simulink model "Main_bikesim_ontest2"  (R2024b)
settings: Solver=FixedStepAuto  StartTime=0.0  StopTime=inf  FixedStep=0.0005
values from neighbouring files (symbols this model uses):
  A_d = permute(A_d,[1,3,2])    [Main_sim.m]    (also in Startup_labview_v2.m; sensor_error_test_sequence.m = (eye(size(A))+Ts*A))
  Ad_t = eye(1)+Ts*A_t    [Main_sim.m]    (also in Startup_labview_v2.m = (eye(size(A_t))+Ts*A_t))
  B_d = zeros(V_n,7,1)    [Main_sim.m]    (also in Startup_labview_v2.m; sensor_error_test_sequence.m = Ts*B)
  badGPS = 0    [Main_sim.m]
  Bd_t = B_t*Ts    [Main_sim.m]    (also in Startup_labview_v2.m)
  bike_model = 1    [Main_sim.m]
  bike_params = LoadBikeParameters(bike)    [Compare_real_to_sim.m]    (also in MPC_Data_train.m = LoadBikeParameters("green"); Main_sim.m; Startup_labview_v2.m; sensor_error_test_sequence.m)
  C = mpc_outer_params.Cd    [MPC_Data_train.m]    (also in Main_sim.m = permute(C,[1,3,2]); Startup_labview_v2.m = permute(C,[1,3,2]); fromIMU2trajectory.m = (W_roll * W_roll.') / max(1, size(W_roll,2)); sensor_data_check.m = (W_roll * W_roll.') / max(1, size(W_roll,2)))
  C_t = zeros(V_n,1)    [Main_sim.m]    (also in Startup_labview_v2.m)
  counter = zeros(V_n,1)    [Main_sim.m]    (also in Startup_labview_v2.m; sensor_error_test_sequence.m = 9)
  D = mpc_outer_params.Dd    [MPC_Data_train.m]    (also in Main_sim.m = zeros(V_n,7,1); Startup_labview_v2.m = zeros(V_n,7,1))
  D_t = zeros(V_n,1)    [Main_sim.m]    (also in Startup_labview_v2.m)
  e1_max = abs(-k2*e2_max/k1)    [Startup_labview_v2.m]
  friction_coefficient = 0.004    [Main_sim.m]
  gg = 9.81    [Main_sim.m]    (also in Startup_labview_v2.m)
  hor_dis = 5    [Main_sim.m]
  I_balancing_outer = 0.0    (= 0)    [Main_sim.m]    (also in Startup_labview_v2.m; sensor_error_test_sequence.m)
  indoor = 0    [Main_sim.m]
  initial_state_estimate = initial_state    [Main_sim.m]    (also in sensor_error_test_sequence.m)
  interpolation = 0    [Main_sim.m]
  k1 = K(1)    [Startup_labview_v2.m]
  k2 = K(2)    [Startup_labview_v2.m]
  K_GPS = permute(K_GPS,[1,3,2])    [Main_sim.m]    (also in Startup_labview_v2.m)
  K_noGPS = permute(K_noGPS,[1,3,2])    [Main_sim.m]    (also in Startup_labview_v2.m)
  lambda = bike_params.lambda    [MPC_Data_train.m]    (also in sensor_error_test_sequence.m = bike_params.lambda_mod)
  lf = bike_params.lf    [MPC_Data_train.m]    (also in sensor_error_test_sequence.m = bike_params.lf_mod)
  linearizedMatrices = [Ad_t, Bd_t, C_t, D_t, V']    [Main_sim.m]
  lr = bike_params.lr    [MPC_Data_train.m]    (also in sensor_error_test_sequence.m = bike_params.lr_mod)
  P_balancing_inner = 3.5    [Main_sim.m]    (also in Startup_labview_v2.m; sensor_error_test_sequence.m)
  P_balancing_outer = 3.75    [Main_sim.m]    (also in Startup_labview_v2.m; sensor_error_test_sequence.m)
  psiref = zeros(length(Xref), 1)    [Refgeneration_test.m]
  ref_dis = 1    [Main_sim.m]    (also in differenttest.m = 0.8; differenttest_Simon.m = 0.1)
  T = [ 1,  sin(phi)*tan(th),  cos(phi)*tan(th) ... (first row only)    [Copy_of_fromIMU2trajectory.m]    (also in Main_sim.m = TransMatrix(bike_params); fromIMU2trajectory.m; sensor_error_test_sequence.m = Rz*Ry*Rx; shorttrajectory.m = table(Xref, Yref, Psiref, Vref, t, 'VariableNames', {'Xref',)
  t_ref = equal_distances / speed    [differenttest.m]    (also in differenttest_Simon.m = linspace(0, (lL-1)/Vref_test, lL)')
  Ts = 0.01    [Main_sim.m]    (also in Startup_labview_v2.m; sensor_error_test_sequence.m)
  V = round(V,1)    [Main_sim.m]    (also in Startup_labview_v2.m)
  v_init = Vref(1)    [Main_sim.m]    (also in Startup_labview_v2.m)
  Vref = zeros(length(Xref), 1)    [Refgeneration_test.m]    (also in differenttest.m = Vref_test * ones(N_line, 1); differenttest_Simon.m = Vref_test * ones(N_line, 1))
  vv = 2.6    [Main_sim.m]    (also in Refgeneration.m = table_ref.v)
  Xref = [Xref;Xref2]    [ReferenceGenerator.m]    (also in concatenate.m; differenttest.m = Xref(:); differenttest_Simon.m = interp1(s, x_path, s_eq, 'linear')')
  Yref = [Yref;Yref2]    [ReferenceGenerator.m]    (also in concatenate.m; differenttest.m = Yref(:); differenttest_Simon.m = interp1(s, y_path, s_eq, 'linear')')
undefined symbols (not defined in the file or in its folder): initial_state, pert_deltadot_state, pert_deltadot_state_fun, pert_phidot_state, pert_phidot_state_fun
libraries: simulink x11, slpidlib x4, matrix_library x1, eeGeneralControl x1
(part 2 of 2)

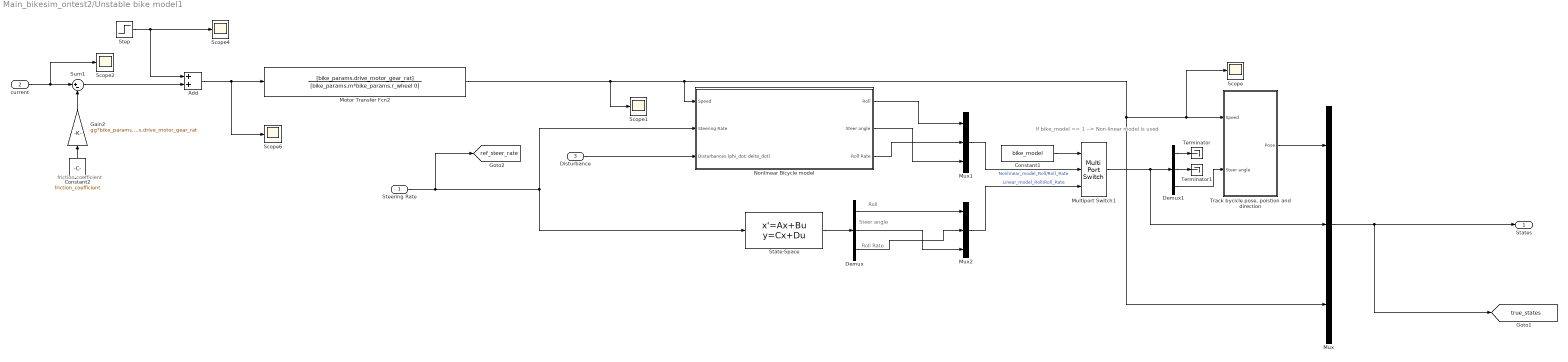
== system Main_bikesim_ontest2/Unstable bike model1 ==
  note: Steer angle
  note: Roll Rate
  note: Roll
  note: If bike_model == 1 --> Non-linear model is used
  note: friction coefficient
  Steering Rate : Inport
  current : Inport  Port=2
  Disturbance : Inport  Port=3
  Add : Sum
  Constant1 : Constant  Value=bike_model
  Constant2 : Constant  Value=friction_coefficient
  Demux : Demux  Outputs=3
  Demux1 : Demux  Outputs=3
  Gain2 : Gain  Gain=gg*bike_params.m*bike_params.r_wheel/bike_params.drive_motor_gear_rat
  Motor Transfer Fcn2 : TransferFcn  Numerator=[bike_params.drive_motor_gear_rat]  Denominator=[bike_params.m*bike_params.r_wheel 0]
  Multiport Switch1 : MultiPortSwitch  Inputs=2  SaturateOnIntegerOverflow=off  InputSameDT=off
  Mux : Mux  Inputs=3
  Mux1 : Mux  Inputs=3
  Mux2 : Mux  Inputs=3
  Nonlinear Bicycle model : Subsystem
  Scope{,1..2,4,6} (5 alike) : Scope
  State-Space : StateSpace  A=[0 0 1; 0 0 0 ; gg/bike_params.h (vv^2/bike_params.h-(gg*bike_params.lr*bike_params.c/(bike_params.h^2*(bike_params.lr+bike_params.lf))))*sin(bike_params.lambda) 0]  B=[0; 1 ; bike_params.lr*vv/((bike_params.lr+bike_params.lf)*bike_params.h)]  C=[1 0 0; 0 1 0 ; 0 0 1]  D=[0;0;0]  InitialCondition=[0; 0 ; 0]
  Step : Step  Time=10  After=0  SampleTime=5
  Sum1 : Sum  Inputs=|+-
  Terminator : Terminator
  Terminator1 : Terminator
  "Track bycicle pose, poistion and direction" : Subsystem
  States : Outport
  tag scope: ref_steer_rate=global, true_states=global
  wires:
  Steering Rate/1 -> State-Space/1, Nonlinear Bicycle model/2(Steering Rate), [ref_steer_rate]
  Nonlinear Bicycle model/3(Roll Rate) -> Mux1/2
  Nonlinear Bicycle model/2(Steer angle) -> Mux1/3
  Demux/1 -> Mux2/1
  Demux/3 -> Mux2/2
  Mux1/1 -> Multiport Switch1/2  "Nonlinear_model_Roll/Roll_Rate"
  Mux2/1 -> Multiport Switch1/3  "Linear_model_Roll/Roll_Rate"
  Constant1/1 -> Multiport Switch1/1
  Disturbance/1 -> Nonlinear Bicycle model/3(Disturbances (phi_dot; delta_dot))
  "Track bycicle pose, poistion and direction"/1(Pose) -> Mux/1
  Mux/1 -> States/1, [true_states]
  Nonlinear Bicycle model/1(Roll) -> Mux1/1
  State-Space/1 -> Demux/1
  Demux/2 -> Mux2/3
  Multiport Switch1/1 -> Mux/2, Demux1/1
  Demux1/3 -> "Track bycicle pose, poistion and direction"/2(Steer angle)
  Demux1/1 -> Terminator/1
  Demux1/2 -> Terminator1/1
  Constant2/1 -> Gain2/1
  Gain2/1 -> Sum1/2
  Sum1/1 -> Add/2
  Motor Transfer Fcn2/1 -> Mux/3, Scope/1, "Track bycicle pose, poistion and direction"/1(Speed), Nonlinear Bicycle model/1(Speed), Scope1/1
  Step/1 -> Add/1, Scope4/1
  current/1 -> Scope2/1, Sum1/1
  Add/1 -> Motor Transfer Fcn2/1, Scope6/1

== system Main_bikesim_ontest2/delta_ref_error ==
  traj_erroe_params : Inport
  e1 : Inport  Port=2
  e2 : Inport  Port=3
  Controller : MATLAB Function  TreatAsAtomicUnit=on
  Integrator : Integrator
  delta_referror : Outport
  wires:
  Controller/1(delta_ref_error) -> delta_referror/1
  e1/1 -> Integrator/1, Controller/3(e1)
  e2/1 -> Controller/4(e2)
  traj_erroe_params/1 -> Controller/1(traj_error_params)
  Integrator/1 -> Controller/2(e1_inte)

== system Main_bikesim_ontest2/delta_ref_psi ==
  Vest : Inport
  d_psiref : Inport  Port=2
  Constant5 : Constant  Value=interpolation
  Constant7 : Constant  Value=linearizedMatrices  VectorParams1D=off
  Delay : Delay  DelayLength=1  SampleTime=Ts
  Filter : MATLAB Function  TreatAsAtomicUnit=on
  To Workspace3 : ToWorkspace  VariableName=delta_psi  SaveFormat=Timeseries  SampleTime=-1
  delta_refpsi : Outport
  wires:
  Delay/1 -> Filter/5(x)
  Constant5/1 -> Filter/4(interpolation)
  Constant7/1 -> Filter/3(linearizedMatrices)
  Vest/1 -> Filter/2(Vest)
  Filter/2(x_dot) -> Delay/1
  Filter/1(delta_ref_psi) -> To Workspace3/1, delta_refpsi/1
  d_psiref/1 -> Filter/1(dpsiref)

== system Main_bikesim_ontest2/Sensors1/Constant disturbances ==
  note: Apply the constant noise after 8sec
  Noise Channel : Inport
  Clock : Clock
  Constant4 : Constant  Value=[1 0.5 -0.2 0.2 0.1 0.02 0.3]'
  Constant7 : Constant  Value=[ 0 0 0 0 0 0 0]
  Create Diagonal Matrix : matrix_library/Create Diagonal Matrix
      settings: LibrarySourceBlock=|
      | simulink/Matrix
      | Operations/Create Diagonal
      | Matrix
  Matrix Multiply : Product  Multiplication=Matrix(*)
  Switch : Switch  Criteria=u2 > Threshold  Threshold=8  SaturateOnIntegerOverflow=off  InputSameDT=off
  Noise : Outport
  wires:
  Create Diagonal Matrix/1 -> Matrix Multiply/1
  Constant7/1 -> Switch/3
  Matrix Multiply/1 -> Switch/1
  Clock/1 -> Switch/2
  Constant4/1 -> Matrix Multiply/2
  Switch/1 -> Noise/1
  Noise Channel/1 -> Create Diagonal Matrix/1

== system Main_bikesim_ontest2/Sensors1/Subsystem ==
  X_coordinate : Inport
  Clock : Clock
  Gain1 : Gain  Gain=badGPS
  Memory : Memory
  Switch : Switch  Criteria=u2 > Threshold  SaturateOnIntegerOverflow=off  InputSameDT=off
  X_coordinate from GPS : Outport
  wires:
  Memory/1 -> Switch/1
  Clock/1 -> Gain1/1
  Switch/1 -> X_coordinate from GPS/1, Memory/1
  Gain1/1 -> Switch/2
  X_coordinate/1 -> Switch/3

== system Main_bikesim_ontest2/Sensors1/Subsystem1 ==
  Y_coordinate : Inport
  Clock : Clock
  Gain1 : Gain  Gain=badGPS
  Memory : Memory
  Switch : Switch  Criteria=u2 > Threshold  SaturateOnIntegerOverflow=off  InputSameDT=off
  Y_coordinate from GPS : Outport
  wires:
  Y_coordinate/1 -> Switch/3
  Gain1/1 -> Switch/2
  Switch/1 -> Memory/1, Y_coordinate from GPS/1
  Clock/1 -> Gain1/1
  Memory/1 -> Switch/1

== system Main_bikesim_ontest2/Unstable bike model1/Nonlinear Bicycle model ==
  Speed : Inport
  Steering Rate : Inport  Port=2
  Disturbances (phi_dot; delta_dot) : Inport  Port=3
  Demux : Demux  Outputs=3
  Integrator2 : Integrator  InitialCondition=[initial_state.roll ; initial_state.steering ; initial_state.roll_rate]
  MATLAB Function : MATLAB Function  TreatAsAtomicUnit=on
  Real Bike Parameters : Constant  Value=[gg bike_params.h bike_params.lr bike_params.lf bike_params.lambda bike_params.c bike_params.m bike_params.IMU_height bike_params.Xgps bike_params.Ygps bike_params.Hgps]  SampleTime=Ts
  Roll : Outport  VectorParamsAs1DForOutWhenUnconnected=off
  Steer angle : Outport  Port=2  VectorParamsAs1DForOutWhenUnconnected=off
  Roll Rate : Outport  Port=3  VectorParamsAs1DForOutWhenUnconnected=off
  wires:
  Steering Rate/1 -> MATLAB Function/2(Steering_rate)
  Disturbances (phi_dot; delta_dot)/1 -> MATLAB Function/4(disturbances)
  Real Bike Parameters/1 -> MATLAB Function/5(bike_params)
  Speed/1 -> MATLAB Function/3(Speed)
  Demux/1 -> Roll/1  "Roll Angle"
  Demux/3 -> Roll Rate/1  "Roll Rate"
  Demux/2 -> Steer angle/1  "Steering Angle"
  Integrator2/1 -> MATLAB Function/1(States), Demux/1
  MATLAB Function/1(xdot) -> Integrator2/1

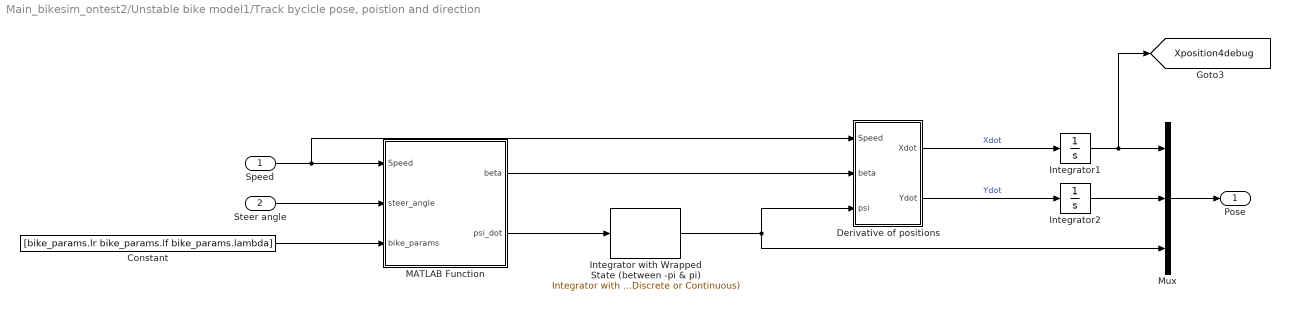
== system Main_bikesim_ontest2/Unstable bike model1/Track bycicle pose, poistion and direction ==
  Speed : Inport
  Steer angle : Inport  Port=2
  Constant : Constant  Value=[bike_params.lr bike_params.lf bike_params.lambda]
  Derivative of positions : MATLAB Function  TreatAsAtomicUnit=on
  Integrator with Wrapped State (between -pi & pi) : eeGeneralControl/Integrator with Wrapped State (Discrete or Continuous)  LabelModeActiveChoice=Discrete  WrappedStateUpperValue=pi  WrappedStateLowerValue=-pi  x0=initial_state_estimate.heading  Ts=Ts
  Integrator1 : Integrator  InitialCondition=initial_state_estimate.x
  Integrator2 : Integrator  InitialCondition=initial_state_estimate.y
  MATLAB Function : MATLAB Function  TreatAsAtomicUnit=on
  Mux : Mux  Inputs=3
  Pose : Outport
  tag scope: Xposition4debug=global
  wires:
  Derivative of positions/2(Ydot) -> Integrator2/1  "Ydot"
  Steer angle/1 -> MATLAB Function/2(steer_angle)
  Integrator2/1 -> Mux/2
  Mux/1 -> Pose/1
  Derivative of positions/1(Xdot) -> Integrator1/1  "Xdot"
  Speed/1 -> MATLAB Function/1(Speed), Derivative of positions/1(Speed)
  Integrator1/1 -> [Xposition4debug], Mux/1
  MATLAB Function/1(beta) -> Derivative of positions/2(beta)
  Constant/1 -> MATLAB Function/3(bike_params)
  MATLAB Function/2(psi_dot) -> Integrator with Wrapped State (between -pi & pi)/1
  Integrator with Wrapped State (between -pi & pi)/1 -> Derivative of positions/3(psi), Mux/3

== matlab function Main_bikesim_ontest2/current position on the trajectory, projection from estimated position ==
  settings: updateMethod=DISCRETE  sampleTime=Ts
  data: Xest input; Yest input; Xref_loc input; Yref_loc input; closest_point input; X_projection output; Y_projection output; closest2closestplus1 output
function [X_projection, Y_projection,closest2closestplus1] = Closest2estOntoClosest2interp(Xest, Yest, Xref_loc, Yref_loc, closest_point)
    
    % Construct vector closest2est
    closest2est = [Xest - Xref_loc(closest_point), Yest - Yref_loc(closest_point)];

    % Construct vector closest2closestplus1
    closest2closestplus1 = [Xref_loc(closest_point+1) - Xref_loc(closest_point), Yref_loc(closest_point+1) - Yref_loc(closest_point)];

    % Calculate the dot product of closest2est and closest2closestplus1
    dot_product = dot(closest2est, closest2closestplus1);

    % Calculate the magnitude squared of closest2closestplus1
    closest2closestplus1_magnitude_squared = dot(closest2closestplus1, closest2closestplus1);

    % Calculate the projection_ratio
    projection_ratio = dot_product/closest2closestplus1_magnitude_squared;

    % Calculate the X coordinate of the projection point
    X_projection = Xref_loc(closest_point) +  projection_ratio*(Xref_loc(closest_point+1) - Xref_loc(closest_point));

    % Calculate the Y coordinate of the projection point
    Y_projection = Yref_loc(closest_point) +  projection_ratio*(Yref_loc(closest_point+1) - Yref_loc(closest_point));
end

== matlab function Main_bikesim_ontest2/Sensors1/MATLAB Function ==
  data: V parameter; C3 output; C parameter; Estimated_Velocity input; interpolation parameter
function C3=fcn(V, C, Estimated_Velocity, interpolation)
% Finding the index of closest and second closest velocities in the calculated velocity vector(in main.m) that corresponds to the
% gains and matrices based on our estimated velocity (i.e the estimated
% velocity is between these two closest V's)
    differences = abs(V - Estimated_Velocity);
    [~, index1] = min(differences);
    differences(index1)=inf;
    [~, index2] = min(differences);

% Implementing linear interpolation when estimated velocity is inside the
% range of minimum and maximum calculated velocity vector
if Estimated_Velocity<=max(V) & Estimated_Velocity>=min(V) & interpolation
    C1=C(index1,:,:);
    C2=C(index2,:,:);
    C1=squeeze(C1);
    C2=squeeze(C2);
    C3=C2*abs((Estimated_Velocity-V(index1))/(V(index1)-V(index2)))+C1*abs((Estimated_Velocity-V(index2))/(V(index1)-V(index2)));
    C3=C3';
    
% If no interpolation or the estimated velocity outside the velocity vector range, then take the closest velocity's gains and matrices
else


    C=C(index1,:,:);
    C3=squeeze(C);
    C3=C3';
end

== matlab function Main_bikesim_ontest2/Trajectory controller + closest_point selection1/Trajectory controller ==
  settings: updateMethod=DISCRETE  sampleTime=Ts
  data: closestpoint_idx_in input; closestpoint_idx_in output; e1 output; e2 output; Xref_loc input; Yref_loc input; psiref_loc input; X_est input; Y_est input; psi_est input; traj_control_params input; v input; Vest input; delta_ref output; delta_ref_psi output; D_psiref output; x input; x_dot output; Ad_t parameter; Bd_t parameter; C_t parameter; D_t parameter; V parameter; interpolation parameter
function [closestpoint_idx_in,e1,e2,delta_ref,delta_ref_psi,D_psiref,x_dot]= ...
    fcn(closestpoint_idx_in,Xref_loc,Yref_loc,psiref_loc,X_est,Y_est,psi_est,traj_control_params, ...
                                                                              v, Vest, x, Ad_t, Bd_t, C_t, D_t, V, interpolation)
%% calculations on a local part of the trajectory

% Unpack parameters, TODO use unpack...
%% qianlei 1023
% gg  = bike_params(1);
% lr = bike_params(2);
% lf = bike_params(3);
% lambda = bike_params(4);

k1 = traj_control_params(1);
k2 = traj_control_params(2);
e1_max = traj_control_params(3);

% Search for closest point --> Finding the closest point going forward. Stop searching once next distance increases
while (Xref_loc(closestpoint_idx_in,1)-X_est)^2 + (Yref_loc(closestpoint_idx_in,1)-Y_est)^2 >= (Xref_loc(closestpoint_idx_in+1,1)-X_est)^2+(Yref_loc(closestpoint_idx_in+1,1)-Y_est)^2  && closestpoint_idx_in <= length(Xref_loc)-2
    closestpoint_idx_in = closestpoint_idx_in+1;
end

% Select same closest point (for heading error and position error)
closestpoint_heading_idx = closestpoint_idx_in;

% Calculate X and Y distance from current location to selected closest
% point
dx = X_est - Xref_loc(closestpoint_idx_in,1);
dy = Y_est - Yref_loc(closestpoint_idx_in,1);

% Calculate difference in current heading and heading in reference point 
% And limit D_psiref  between pi and -pi
D_psiref = psiref_loc(closestpoint_idx_in+1,1)-psiref_loc(closestpoint_idx_in,1);
D_psiref = wrapToPi(D_psiref);
% if D_psiref>=pi
%     D_psiref=mod(D_psiref,-2*pi);
% end
% if D_psiref<=-pi
%     D_psiref=mod(D_psiref,2*pi);
% end

%IMPROVEMENT: implement an interpolation algoritm
% Calculate distence between point before closest point and current location
dist_true_previous = sqrt((Xref_loc(closestpoint_idx_in-1,1)-X_est)^2+(Yref_loc(closestpoint_idx_in-1,1)-Y_est)^2);
% Angle of line between previous closest point and current location
alpha_star = atan((Yref_loc(closestpoint_idx_in-1,1)-Y_est)/(Xref_loc(closestpoint_idx_in-1,1)-X_est));
% heading previous closest point - alpha star
alpha_projected_dist = alpha_star-psiref_loc(closestpoint_idx_in,1);
% the distance from the previous closest point to the projection of the bike on the trajectory
Projected_dist = abs(dist_true_previous*cos(alpha_projected_dist));

compared_dist = sqrt((Xref_loc(closestpoint_idx_in,1)-Xref_loc(closestpoint_idx_in-1,1))^2+(Yref_loc(closestpoint_idx_in,1)-Yref_loc(closestpoint_idx_in-1,1))^2);

% If bike passes closest point, the heading of the next point will be taken
if Projected_dist >= compared_dist
closestpoint_heading_idx = closestpoint_idx_in+1;
end

%calculate e1 and e2        
e1= dy*cos(psiref_loc(closestpoint_heading_idx,1)) - dx*sin(psiref_loc(closestpoint_heading_idx,1)); % this make e1 include "direction" automatically
e2= psi_est-psiref_loc(closestpoint_heading_idx,1); %calculate e2

% closest point on the local trajectory
ref_X=Xref_loc(closestpoint_idx_in,1);
ref_Y=Yref_loc(closestpoint_idx_in,1);
ref_psi=psiref_loc(closestpoint_heading_idx,1);

 % keep heading error should be between -pi 2 pi
e2 = wrapToPi(e2);
%e2=mod(e2+pi,2*pi)-pi;     

% Steering contribution from trajectory error
% delta_ref_error=-k1*sign(e1)*min(abs(e1),e1_max)-k2*e2;
delta_e1 = -k1*sign(e1)*min(abs(e1),e1_max);
delta_e2 =-k2*e2;
% delta_e1 = -2;
% delta_e2 = 0;
%delta_ref_error = delta_e1 + delta_e2;

% Steering contribution from trajectory error, ie feedback of trajectory
% error
delta_ref_error = -k1*sign(e1)*min(abs(e1),e1_max)-k2*e2;

% the following lines is a filtering of the reference direction, it is
% a speed dependent linear filter

% TODO is similar interpolations done on other places, for example in the
% Kalman filter_ If yes, check if a common function can be used and avoid
% doubling code

%calculate the time between psiref(idx,1) and psiref(idx+1,1)
dX=Xref_loc(closestpoint_idx_in+1,1)-ref_X;
dY=Yref_loc(closestpoint_idx_in+1,1)-ref_Y;
dis=sqrt(dX^2+dY^2);
Ts_psi=dis/v;

% Sample dpsiref
dpsiref=(D_psiref)/Ts_psi;


% Finding the index of closest and second closest velocities in the calculated velocity vector(in main.m) that corresponds to the
% gains and matrices based on our estimated velocity (i.e the estimated
% velocity is between these two closest V's)
differences = abs(V - Vest);
[~, index1] = min(differences);
differences(index1)=inf;
[~, index2] = min(differences);

% Implementing linear interpolation when estimated velocity is inside the
% range of minimum and maximum calculated velocity vector
if Vest<=max(V) & Vest>=min(V) & interpolation

    Ad_t1=Ad_t(index1,:);
    Ad_t2=Ad_t(index2,:);
    Ad_t=Ad_t2*abs((Vest-V(index1))/(V(index1)-V(index2)))+Ad_t1*abs((Vest-V(index2))/(V(index1)-V(index2)));
    Bd_t1=Bd_t(index1,:);
    Bd_t2=Bd_t(index2,:);
    Bd_t=Bd_t2*abs((Vest-V(index1))/(V(index1)-V(index2)))+Bd_t1*abs((Vest-V(index2))/(V(index1)-V(index2)));
    C_t1=C_t(index1,:);
    C_t2=C_t(index2,:);
    C_t=C_t2*abs((Vest-V(index1))/(V(index1)-V(index2)))+C_t1*abs((Vest-V(index2))/(V(index1)-V(index2)));
    D_t1=D_t(index1,:);
    D_t2=D_t(index2,:);
    D_t=D_t2*abs((Vest-V(index1))/(V(index1)-V(index2)))+D_t1*abs((Vest-V(index2))/(V(index1)-V(index2)));
    
% If no interpolation or the estimated velocity outside the velocity vector range, then take the closest velocity's gains and matrices
else
    Ad_t=Ad_t(index1,:);
    Bd_t=Bd_t(index1,:);
    C_t=C_t(index1,:);
    D_t=D_t(index1,:);
end


% Steering contribution from heading change
x_dot = Ad_t*x + Bd_t*dpsiref;
delta_ref_psi = (C_t*x + D_t*dpsiref); 
% delta_ref_psi = 0; 

% Total steering reference 
delta_ref = delta_ref_psi + delta_ref_error;

% limit steer angle between -pi/4 and pi/4
if delta_ref>=pi/4
    delta_ref=pi/4;
end

if delta_ref<=-pi/4
    delta_ref=-pi/4;
end

% % Transform steering reference into roll reference for balancing controller
% eff_delta_ref = delta_ref*sin(lambda);
% roll_ref = -1*atan(tan(eff_delta_ref)*(Vest^2/(lr+lf))/gg);

end

== matlab function Main_bikesim_ontest2/   ==
  settings: updateMethod=DISCRETE  sampleTime=Ts
  data: delta_ref input; roll_ref output; Vest input; bike_params input
function roll_ref  = fcn(delta_ref, Vest, bike_params)

gg  = bike_params(1);
lr  = bike_params(2);
lf  = bike_params(3);
lambda = bike_params(4);

%% Transform steering reference into roll reference for balancing controller
% this is done using the static relation between steering angle and roll,
% ie the relatin you have if the bike is constantly being in a circle
eff_delta_ref = delta_ref*sin(lambda);
roll_ref = -1*atan(tan(eff_delta_ref)*(Vest^2/(lr+lf))/gg);

end

== matlab function Main_bikesim_ontest2/Sensors1/Define true sensor positions on the bike ==
  data: bike_params input; pose input; pose_corrected output
function pose_corrected  = fcn(bike_params, pose)
pose_corrected = pose;

gpsX = bike_params(1); % measured offset of GPS parallel to bike
gpsY = bike_params(2); % measured offset of GPS perpendicular to bike
gpsH = bike_params(3); % measured offset of GPS from ground to GPS

% define pose_l
pose_l = pose;

% Transform to local frame
    pose_l(1) =  pose(1) * cos(pose(3)) + pose(2) * sin(pose(3));
    pose_l(2) = -pose(1) * sin(pose(3)) + pose(2) * cos(pose(3)); 

% define actual positions of GPS 
% pose1 = difference in x in local frame
% pose2 = difference in y in local frame
    pose_l(1) = pose_l(1) + gpsX;
    pose_l(2) = pose_l(2) + gpsY + gpsH*sin(pose(4));

% define actual positions of IMU 


% Transform back to global frame
    pose(1) = pose_l(1) * cos(pose(3)) - pose_l(2) * sin(pose(3));
    pose(2) = pose_l(1) * sin(pose(3)) + pose_l(2) * cos(pose(3));

pose_corrected(1) = pose(1);
pose_corrected(2) = pose(2);

== matlab function Main_bikesim_ontest2/reference position at time t, interpolation of reference points  ==
  settings: updateMethod=DISCRETE  sampleTime=Ts
  data: Xref_t output; Yref_t output; Xref_loc input; Yref_loc input; t_ref_loc input; vref_loc input; t_now input; vref_t output
function [Xref_t,Yref_t,vref_t]= fcn(Xref_loc,Yref_loc,t_ref_loc,vref_loc,t_now) 
    
disp(t_now)
disp([Xref_loc Yref_loc t_ref_loc])
    % Find index point before the bike
    n = 1; 
    
    if t_now < t_ref_loc(1)
        disp('this should not happen, check reference point in position controller');
    end

    %% 
    while t_now >= t_ref_loc(n+1), n = n+1;end  
    
    % Calculate normalized time ratio between two reference points
    t_int=(t_now-t_ref_loc(n))/(t_ref_loc(n+1)-t_ref_loc(n)); 
       
    % X_ref position at t_now using linear interpolation between n and n+1
    Xref_t = Xref_loc(n)+t_int*(Xref_loc(n+1)-Xref_loc(n));   

    % Y_ref position at t_now using linear interpolation between n and n+1
    Yref_t = Yref_loc(n)+t_int*(Yref_loc(n+1)-Yref_loc(n));    

    % v_ref position at t_now using linear interpolation between n and n+1
    vref_t = vref_loc(n)+t_int*(vref_loc(n+1)-vref_loc(n));

end

== matlab function Main_bikesim_ontest2/State estimator1/Linearized Bicycle Model on Constant Velocity ==
  data: Est_States input; dot_delta input; y input; bike_params input; Est_states output; flag input; T parameter; indoor parameter; K_GPS parameter; K_noGPS parameter; V parameter; A_d parameter; B_d parameter; C parameter; D parameter; interpolation parameter
function Est_states  = fcn(Est_States, dot_delta, y, bike_params, flag, T, indoor, K_GPS, K_noGPS, V, A_d, B_d, C, D, interpolation)
% description 
% Inputs
%   Est_States := [X Y psi phi phi_dot delta v] are global at time t 
%   dot_delta_e := effective steering rate
%   y := measurement vector
%   bike_params := vector of bike parameters + gravity
%   flag := [0-1] increasing counter reseted at 1. When flag == 0 means
%           that GPS measurement is available
%   indoor := it's 1 when you want to run the bike indoor
%   K_GPS := Computed state_feedback gain including GPS meas
%   K_noGPS := Computed state_feedback gain excluding GPS meas
%
% Outputs
%   Est_states : = [X Y psi phi phi_dot delta v] global at time t+1

% PROBABLY IS BETTER IF WE CHANGE THE NAME OF Est_states AND Est_States

% Transform the states to local frame 
    Est_States_l = zeros(7,1);
    
    Est_States_l(1) = Est_States(1) * cos(Est_States(3)) + Est_States(2) * sin(Est_States(3));
    Est_States_l(2) = -Est_States(1) * sin(Est_States(3)) + Est_States(2) * cos(Est_States(3));
    Est_States_l(3) = 0;        % direction of bike is aligned with X local frame
    Est_States_l(4) = Est_States(4);
    Est_States_l(5) = Est_States(5);
    Est_States_l(6) = Est_States(6);
    Est_States_l(7) = Est_States(7);

% Transform measurements to local frame
    y_l = zeros(size(y));

    y_l(1) = y(1) * cos(Est_States(3)) + y(2) * sin(Est_States(3));
    y_l(2) = -y(1) * sin(Est_States(3)) + y(2) * cos(Est_States(3)); 
    % y_l(3) = y(3);
    % y_l(4) = y(4);
    % y_l(5) = y(5);
    % y_l(6) = y(6);
    % y_l(7) = y(7);
    y_l(3:7) = y(3:7);

% Correct for parameter values/sensor positions
% The parameters/positions are measures by us (can differ from true values)
    X_gps_mod = bike_params(1);
    Y_gps_mod = bike_params(2);
    H_gps_mod = bike_params(3);
    
    y_l(1) = y_l(1) - X_gps_mod;
    y_l(2) = y_l(2) - Y_gps_mod - H_gps_mod*sin(Est_States(4));
    
% IMU correction
    raw_acc  = [0 y_l(3) 0];
    raw_gyro = [y_l(4) 0 y_l(5)];
    
% Apply the correction to the accelerometer measurement
    acc_corr = T*raw_acc';
    
% Apply the correction to the gyro measurement
    gyro_corr = T*raw_gyro';
% Results
    y_l(3) =acc_corr(2) ;
    y_l(4) =gyro_corr(1) ;
    y_l(5) =gyro_corr(3) ;
    % 
% % Continuous Time update in local frame TODO: x(t+1) = (I+A delta_T)h_hat(t)
    %     states_dot = zeros(7,1);
    %     
    %     states_dot(1) = Est_States(7);
    %     states_dot(2) = v * (Est_States_l(3) + (lr/(lr+lf))*Est_States(6) );
    %     states_dot(3) = (v/(lr+lf)) * Est_States(6);
    %     states_dot(4) = Est_States(5);
    %     states_dot(5) =(g/h)*Est_States(4) + ((lr*v)/((lr+lf)*h))*sin(lambda)*dot_delta + ((h*v^2-g*lr*c)/((lr+lf)*h^2))*sin(lambda)*Est_States(6);
    %     states_dot(6) = dot_delta;
    %     states_dot(7) = 0;
    % 
% % Discrete time update in local 
    %     Est_States_l = Est_States_l + states_dot * Ts; 
    
% % C identity is used to see if the code runs
    %     sen = zeros(6,1);
    %     sen(1)      = States_l(1);  
    %     sen(2)      = States_l(2);
    %     %sen(3)      = States_l(3);
    %     sen(3)      = States_l(4);
    %     sen(4)      = States_l(5);
    %     sen(5)      = States_l(6);
    %     sen(6)      = States_l(7);
    
% % Transform measurements into local frame to see if code runs
    %     meas_l = zeros(6,1);
    %     meas_l(1) = meas(1) * cos(States(3)) + meas(2) * sin(States(3));
    %     meas_l(2) = -meas(1) * sin(States(3)) + meas(2) * cos(States(3));
    %     meas_l(3) = 0;
    %     meas_l(3) = meas(3)-States(3);  
    %     meas_l(3) = meas(4);
    %     meas_l(4) = meas(5);
    %     meas_l(5) = meas(6);
    %     meas_l(6) = meas(7);
    %     meas_l(7) = meas(7);
%b3rbrgb

% Finding the index of closest and second closest velocities in the calculated velocity vector(in main.m) that corresponds to the
% gains and matrices based on our estimated velocity (i.e the estimated
% velocity is between these two closest V's)
    differences = abs(V - Est_States(7));
    [~, index1] = min(differences);
    differences(index1)=inf;
    [~, index2] = min(differences);

% Implementing linear interpolation when estimated velocity is inside the
% range of minimum and maximum calculated velocity vector
if Est_States(7)<=max(V) & Est_States(7)>=min(V) & interpolation

    K_GPS1=K_GPS(index1,:,:);
    K_GPS2=K_GPS(index2,:,:);
    K_GPS1=squeeze(K_GPS1);
    K_GPS2=squeeze(K_GPS2);
    K_GPS=K_GPS2*abs((Est_States(7)-V(index1))/(V(index1)-V(index2)))+K_GPS1*abs((Est_States(7)-V(index2))/(V(index1)-V(index2)));

    K_noGPS1=K_noGPS(index1,:,:);
    K_noGPS2=K_noGPS(index2,:,:);
    K_noGPS1=squeeze(K_noGPS1);
    K_noGPS2=squeeze(K_noGPS2);
    K_noGPS=K_noGPS2*abs((Est_States(7)-V(index1))/(V(index1)-V(index2)))+K_noGPS1*abs((Est_States(7)-V(index2))/(V(index1)-V(index2)));
   
    Ad1=A_d(index1,:,:);
    Ad2=A_d(index2,:,:);
    Ad1=squeeze(Ad1);
    Ad2=squeeze(Ad2);
    A_d=Ad2.*abs((Est_States(7)-V(index1))/(V(index1)-V(index2)))+Ad1*abs((Est_States(7)-V(index2))/(V(index1)-V(index2)));

    Bd1=B_d(index1,:,:);
    Bd2=B_d(index2,:,:);
    Bd1=squeeze(Bd1);
    Bd2=squeeze(Bd2);
    B_d=Bd2*abs((Est_States(7)-V(index1))/(V(index1)-V(index2)))+Bd1*abs((Est_States(7)-V(index2))/(V(index1)-V(index2)));

    C1=C(index1,:,:);
    C2=C(index2,:,:);
    C1=squeeze(C1);
    C2=squeeze(C2);
    C=C2*abs((Est_States(7)-V(index1))/(V(index1)-V(index2)))+C1*abs((Est_States(7)-V(index2))/(V(index1)-V(index2)));

    D1=D(index1,:,:);
    D2=D(index2,:,:);
    D1=squeeze(D1);
    D2=squeeze(D2);
    D=D2*abs((Est_States(7)-V(index1))/(V(index1)-V(index2)))+D1*abs((Est_States(7)-V(index2))/(V(index1)-V(index2)));

% If no interpolation or the estimated velocity outside the velocity vector range, then take the closest velocity's gains and matrices
else 
    K_GPS=K_GPS(index1,:,:);
    K_GPS=squeeze(K_GPS);

    K_noGPS=K_noGPS(index1,:,:);
    K_noGPS=squeeze(K_noGPS);

    A_d=A_d(index1,:,:);
    A_d=squeeze(A_d);
    B_d=B_d(index1,:,:);
    B_d=squeeze(B_d);
    C=C(index1,:,:);
    C=squeeze(C);
    D=D(index1,:,:);
    D=squeeze(D);
end
% Time update in local frame (from t to t+1)

    % Time update
     Est_States_l = A_d'*Est_States_l + B_d'*dot_delta;

    % Measurement update in local frame
     Est_states_l = zeros(7,1);

    % Sampling differentiation (Sensors rate 100Hz but GPS 10Hz)

    if flag == 0 && indoor == 0 % new GPS measurement and outdoor    
        K = K_GPS';

    else % no new GPS measurement or indoor    
        K = K_noGPS';
    end

% Measurement prediction
    y_pred = C'*Est_States_l + D'*dot_delta;

% Measurement update
    Est_states_l = Est_States_l + K * (y_l - y_pred);
    
    %Useless?
    % states_l = Kalman_gain * (meas_l - sen);
    % states_l(1) = States_l(1) + Kalman_gain(1,1) * (meas_l(1) - x_m) + Kalman_gain(1,2) * (meas_l(2) - y_m) + Kalman_gain(1,3) * (meas_l(3) - psi_m) + Kalman_gain(1,4) * (meas_l(4) - phi_m) + Kalman_gain(1,5) * (meas_l(5) - dot_phi_m) + Kalman_gain(1,6) * (meas_l(6) - delta_m) + Kalman_gain(1,7) * (meas_l(7) - v_m);
    % states_l(2) = States_l(2) + Kalman_gain(2,1) * (meas_l(1) - x_m) + Kalman_gain(2,2) * (meas_l(2) - y_m) + Kalman_gain(2,3) * (meas_l(3) - psi_m) + Kalman_gain(2,4) * (meas_l(4) - phi_m) + Kalman_gain(2,5) * (meas_l(5) - dot_phi_m) + Kalman_gain(2,6) * (meas_l(6) - delta_m) + Kalman_gain(2,7) * (meas_l(7) - v_m);
    % states_l(3) = States_l(3) + Kalman_gain(3,1) * (meas_l(1) - x_m) + Kalman_gain(3,2) * (meas_l(2) - y_m) + Kalman_gain(3,3) * (meas_l(3) - psi_m) + Kalman_gain(3,4) * (meas_l(4) - phi_m) + Kalman_gain(3,5) * (meas_l(5) - dot_phi_m) + Kalman_gain(3,6) * (meas_l(6) - delta_m) + Kalman_gain(3,7) * (meas_l(7) - v_m);
    % states_l(4) = States_l(4) + Kalman_gain(4,1) * (meas_l(1) - x_m) + Kalman_gain(4,2) * (meas_l(2) - y_m) + Kalman_gain(4,3) * (meas_l(3) - psi_m) + Kalman_gain(4,4) * (meas_l(4) - phi_m) + Kalman_gain(4,5) * (meas_l(5) - dot_phi_m) + Kalman_gain(4,6) * (meas_l(6) - delta_m) + Kalman_gain(4,7) * (meas_l(7) - v_m);
    % states_l(5) = States_l(5) + Kalman_gain(5,1) * (meas_l(1) - x_m) + Kalman_gain(5,2) * (meas_l(2) - y_m) + Kalman_gain(5,3) * (meas_l(3) - psi_m) + Kalman_gain(5,4) * (meas_l(4) - phi_m) + Kalman_gain(5,5) * (meas_l(5) - dot_phi_m) + Kalman_gain(5,6) * (meas_l(6) - delta_m) + Kalman_gain(5,7) * (meas_l(7) - v_m);
    % states_l(6) = States_l(6) + Kalman_gain(6,1) * (meas_l(1) - x_m) + Kalman_gain(6,2) * (meas_l(2) - y_m) + Kalman_gain(6,3) * (meas_l(3) - psi_m) + Kalman_gain(6,4) * (meas_l(4) - phi_m) + Kalman_gain(6,5) * (meas_l(5) - dot_phi_m) + Kalman_gain(6,6) * (meas_l(6) - delta_m) + Kalman_gain(6,7) * (meas_l(7) - v_m);
    % states_l(7) = States_l(7) + Kalman_gain(7,1) * (meas_l(1) - x_m) + Kalman_gain(7,2) * (meas_l(2) - y_m) + Kalman_gain(7,3) * (meas_l(3) - psi_m) + Kalman_gain(7,4) * (meas_l(4) - phi_m) + Kalman_gain(7,5) * (meas_l(5) - dot_phi_m) + Kalman_gain(7,6) * (meas_l(6) - delta_m) + Kalman_gain(7,7) * (meas_l(7) - v_m);

% Transform to global the local states at time t+1 after measurement update
    Est_states = zeros(7,1);
    Est_states(3) = Est_States(3) + Est_states_l(3);    % direction update global
    
% Change of Coordinates from local to global frame for  states 
    Est_states(1) = Est_states_l(1) * cos(Est_States(3)) - Est_states_l(2) * sin(Est_States(3));
    Est_states(2) = Est_states_l(1) * sin(Est_States(3)) + Est_states_l(2) * cos(Est_States(3));
    Est_states(4) = Est_states_l(4);
    Est_states(5) = Est_states_l(5);
    Est_states(6) = Est_states_l(6);
    Est_states(7) = Est_states_l(7);


    
% Heading angle between pi and -pi
    Est_states(3) = wrapToPi(Est_states(3));

end

== matlab function Main_bikesim_ontest2/calculate pose_error based on projection point to reference point at time t ==
  settings: updateMethod=DISCRETE  sampleTime=Ts
  data: pose_error output; Xref_t input; Yref_t input; X_projection input; Y_projection input; closest2closestplus1 input
function pose_error  = calculatePoseError(Xref_t, Yref_t, X_projection, Y_projection, closest2closestplus1)
    % Function to calculate pose_error based on projection point to reference point
    
    % Step 1: Create the vector from projection point to reference point
    % This vector points from (X_projection, Y_projection) to (Xref_t, Yref_t)
    projectionpoint2referencepoint = [Xref_t - X_projection, Yref_t - Y_projection];  

    % Step 2: Perform the dot product of the two vectors
    dot_product = dot(projectionpoint2referencepoint, closest2closestplus1);
    
    % Step 3: Calculate the length of the projectionpoint2referencepoint vector
    % The length of the vector is its Euclidean norm
    vector_length = norm(projectionpoint2referencepoint);
    
    % Step 4: Determine pose_error based on the dot product sign
    if dot_product < 0
        pose_error = -vector_length; % Negative length if dot product is negative (ahead of reference point)
    else
        pose_error = vector_length;  % Positive length otherwise (behind reference point)
    end

end

== matlab function Main_bikesim_ontest2/delta_ref_error/Controller ==
  settings: updateMethod=DISCRETE  sampleTime=Ts
  data: traj_error_params input; e1_inte input; e1 input; delta_ref_error output; e2 input
function delta_ref_error = fcn (traj_error_params,e1_inte,e1,e2) 
%% calculations on a local part of the trajectory
k_inte = 0.01; %% Should be removed to outside and it is used for the integration of e1s 
k1 = traj_error_params(1);
k2 = traj_error_params(2);
e1_max = traj_error_params(3);
% Steering contribution from trajectory error
delta_ref_error = -k1*sign(e1)*min(abs(e1),e1_max) - k2*e2 - k_inte * e1_inte;

end

== matlab function Main_bikesim_ontest2/Unstable bike model1/Nonlinear Bicycle model/MATLAB Function ==
  data: States input; xdot output; Steering_rate input; Speed input; disturbances input; bike_params input
function xdot  = fcn(States, Steering_rate, Speed, disturbances, bike_params)
% Unpacked bike_params
    g = bike_params(1);
    h = bike_params(2);
    lr = bike_params(3);
    lf = bike_params(4);
    lambda = bike_params(5);
    c = bike_params(6);
    %m = bike_params(7);
    %h_imu = bike_params(8);

phi =   States(1);%roll
delta = States(2);%steering angle
phi_d = States(3);%rollrate

% xdot = [phidot deltadot phiddot]
xdot1 = phi_d + disturbances(1);
xdot2 = Steering_rate + disturbances(2);
xdot3 = (g/h)*sin(phi) + ((lr*Speed)/((lr+lf)*h))/(cos(sin(lambda)*delta)^2)*sin(lambda)*Steering_rate ...
                                  + ((Speed^2/h)-(g*lr*c/(h^2*(lr+lf))))*sin(lambda)*tan(delta);

% linearized
% xdot3 = (g/h)*phi + ((lr*Speed)/((lr+lf)*h))*Steering_rate + ((Speed^2/h)-(g*lr*c/(h^2*(lr+lf))))*sin(lambda)*delta;

xdot = [xdot1 xdot2 xdot3]';

== matlab function Main_bikesim_ontest2/Nearest point algrithm/   ==
  settings: updateMethod=DISCRETE  sampleTime=Ts
  data: e1 output; e2 output; closestpoint_idx output; closestpoint_heading_idx output; Xref_loc input; Yref_loc input; psiref_loc input; X_est input; Y_est input; psi_est input; ref_X output; ref_Y output; ref_psi output; dpsiref output; Local_Vref input
function [e1,e2,closestpoint_idx,closestpoint_heading_idx,ref_X,ref_Y,ref_psi,dpsiref]= fcn (Xref_loc,Yref_loc,psiref_loc, X_est,Y_est,psi_est,Local_Vref) 
%% calculations on a local part of the trajectory
% Each referencepoint has a location (X,Y) and a heading
% The heading is defined in the startup.m file as 'the heading where its coming from' 
% Second point in local reference is current selected closest point

closestpoint_idx=2;
% Search for closest point
% Finding the closest point going forward. Stop searching once next distance increases

while (Xref_loc(closestpoint_idx,1)-X_est)^2 + (Yref_loc(closestpoint_idx,1)-Y_est)^2 >= (Xref_loc(closestpoint_idx+1,1)-X_est)^2+(Yref_loc(closestpoint_idx+1,1)-Y_est)^2  && closestpoint_idx <= length(Xref_loc)-2
closestpoint_idx = closestpoint_idx+1;
end

% Select same closest point (for heading error and position error)
closestpoint_heading_idx = closestpoint_idx;

% Calculate X and Y distance from current location to selected closest
% point
dx = X_est - Xref_loc(closestpoint_idx,1);
dy = Y_est - Yref_loc(closestpoint_idx,1);
% Calculate difference in current heading and heading in reference point 
% And limit D_psiref  between -2pi and 2pi
D_psiref=psiref_loc(closestpoint_idx+1,1)-psiref_loc(closestpoint_idx,1);
if D_psiref>=pi
    D_psiref=mod(D_psiref,-2*pi);
end
if D_psiref<=-pi
    D_psiref=mod(D_psiref,2*pi);
end
%IMPROVEMENT: implement an interpolation algoritm, why this comment?

% Calculate distence between point before closest point and current location
dist_true_previous = sqrt((Xref_loc(closestpoint_idx-1,1)-X_est)^2+(Yref_loc(closestpoint_idx-1,1)-Y_est)^2);
% Angle of line between previous closest point and current location
alpha_star = atan((Yref_loc(closestpoint_idx-1,1)-Y_est)/(Xref_loc(closestpoint_idx-1,1)-X_est));
% heading previous closest point - alpha star
alpha_projected_dist = alpha_star-psiref_loc(closestpoint_idx,1);
% the distance from the previous closest point to the projection of the bike on the trajectory
Projected_dist = abs(dist_true_previous*cos(alpha_projected_dist));

compared_dist = sqrt((Xref_loc(closestpoint_idx,1)-Xref_loc(closestpoint_idx-1,1))^2+(Yref_loc(closestpoint_idx,1)-Yref_loc(closestpoint_idx-1,1))^2);

% If bike passes closest point, the heading of the next point will be taken
if Projected_dist >= compared_dist
closestpoint_heading_idx = closestpoint_idx+1;
end

%calculate e1 and e2        
e1= dy*cos(psiref_loc(closestpoint_heading_idx,1)) - dx*sin(psiref_loc(closestpoint_heading_idx,1)); % this make e1 include "direction" automatically
e2= psi_est-psiref_loc(closestpoint_heading_idx,1); %calculate e2

% closest point on the local trajectory
ref_X=Xref_loc(closestpoint_idx,1);
ref_Y=Yref_loc(closestpoint_idx,1);
ref_psi=psiref_loc(closestpoint_heading_idx,1);
% keep heading error should be between -pi 2 pi
e2 = wrapToPi(e2);
%e2=mod(e2+pi,2*pi)-pi;    
%calculate the time between psiref(idx,1) and psiref(idx+1,1)
dX=Xref_loc(closestpoint_idx+1,1)-ref_X;
dY=Yref_loc(closestpoint_idx+1,1)-ref_Y;
dis=sqrt(dX^2+dY^2);
Ts_psi=dis/Local_Vref(1);

% Sample dpsiref
dpsiref=(D_psiref)/Ts_psi;

% Reset closest point index as feedback for local frame selection
closestpoint_idx = closestpoint_idx-1;


end

== matlab function Main_bikesim_ontest2/Unstable bike model1/Track bycicle pose, poistion and direction/Derivative of positions ==
  data: Speed input; beta input; psi input; Xdot output; Ydot output
function [Xdot, Ydot]  = fcn(Speed, beta, psi)

Xdot = Speed * cos(psi + beta);
Ydot = Speed * sin(psi + beta);

== matlab function Main_bikesim_ontest2/Unstable bike model1/Track bycicle pose, poistion and direction/MATLAB Function ==
  data: Speed input; steer_angle input; beta output; bike_params input; psi_dot output
function [beta, psi_dot] = fcn(Speed, steer_angle, bike_params)
lr       = bike_params(1);
lf       = bike_params(2);
lambda  = bike_params(3);

eff_steering = steer_angle*sin(lambda);

beta = atan(lr /(lr+lf) * tan(eff_steering) );
psi_dot = (Speed / lr) * sin(beta);

== matlab function Main_bikesim_ontest2/delta_ref_psi/Filter ==
  settings: updateMethod=DISCRETE  sampleTime=Ts
  data: dpsiref input; Vest input; delta_ref_psi output; x_dot output; linearizedMatrices input; interpolation input; x input
function [delta_ref_psi,x_dot]= fcn (dpsiref,Vest, linearizedMatrices,interpolation,x) 
%% calculations on a local part of the trajectory
Ad_t=linearizedMatrices(:,1);
Bd_t=linearizedMatrices(:,2);
C_t=linearizedMatrices(:,3);
D_t=linearizedMatrices(:,4);
VV=linearizedMatrices(:,5)';


% Finding the index of closest and second closest velocities in the calculated velocity vector(in main.m) that corresponds to the
% gains and matrices based on our estimated velocity (i.e the estimated
% velocity is between these two closest V's)
differences = abs(VV - Vest);
[~, index1] = min(differences);
differences(index1)=inf;
[~, index2] = min(differences);

% Implementing linear interpolation when estimated velocity is inside the
% range of minimum and maximum calculated velocity vector
if Vest<=max(VV) && Vest>=min(VV) && interpolation

    Ad_t1=Ad_t(index1,:);
    Ad_t2=Ad_t(index2,:);
    Ad_t=Ad_t2*abs((Vest-VV(index1))/(VV(index1)-VV(index2)))+Ad_t1*abs((Vest-VV(index2))/(VV(index1)-VV(index2)));
    Bd_t1=Bd_t(index1,:);
    Bd_t2=Bd_t(index2,:);
    Bd_t=Bd_t2*abs((Vest-VV(index1))/(VV(index1)-VV(index2)))+Bd_t1*abs((Vest-VV(index2))/(VV(index1)-VV(index2)));
    C_t1=C_t(index1,:);
    C_t2=C_t(index2,:);
    C_t=C_t2*abs((Vest-VV(index1))/(VV(index1)-VV(index2)))+C_t1*abs((Vest-VV(index2))/(VV(index1)-VV(index2)));
    D_t1=D_t(index1,:);
    D_t2=D_t(index2,:);
    D_t=D_t2*abs((Vest-VV(index1))/(VV(index1)-VV(index2)))+D_t1*abs((Vest-VV(index2))/(VV(index1)-VV(index2)));

% If no interpolation or the estimated velocity outside the velocity vector range, then take the closest velocity's gains and matrices
else
    Ad_t=Ad_t(index1,:);
    Bd_t=Bd_t(index1,:);
    C_t=C_t(index1,:);
    D_t=D_t(index1,:);
end

% Steering contribution from heading change
x_dot = Ad_t*x + Bd_t*dpsiref;
delta_ref_psi = C_t*x + D_t*dpsiref; 

end

== matlab function Main_bikesim_ontest2/Selection of local reference from total reference1/Local reference selection & stop funcion ==
  data: last_ids input; ids output; xref input; local_Xref output size=Nn [..30000]; local_Yref output size=Nn [..30000]; local_Psiref output size=Nn [..30000]; local_Vref output size=Nn; local_tref output size=Nn; yref input; psiref input; Vref input; closest_point input; tref input; ref_dis parameter; hor_dis parameter; stop output; abort input; est input
function [ids,local_Xref,local_Yref,local_Psiref,local_Vref,local_tref,stop] = fcn(last_ids,xref,yref,psiref,Vref, closest_point, tref, ref_dis, hor_dis,abort,est)
% Local reference trajectory starts at point before the current closest
% point and has a length of M
ids=last_ids+closest_point-1;      % calculate the initial index of the points that will be sent to next block (first point of local_ref)

Ns=ceil(hor_dis/ref_dis);          % hor_dis, ref_dis are definited in "StudentProject2021.m", Ns is the length of the local trajectory sent to next block
M=ids+Ns;                          % calculate the end index of the local reference
n=size(xref,1);                    % length of whole trajectory  

if M>n                             % if reached near end of reference, local trajectry becomes shorter
    M=n;
    disp('Bike position close to end of reference so that local reference partly beyoined the reference.'); 
end

% Temporary simulation STOP to prevent singularity error once approaching
% the end of the trajectory
% Simulation stops before the end of the reference trajectory
stop = 0;
if ids >= n-ceil(n/20)
    stop = 1;
    disp('Bike close to end of trajectory.');
end


% Start always at second value of total reference
if ids<2
ids = 2;
end

% Select local reference from total reference
local_Xref = xref(ids-1:M,1);
local_Yref = yref(ids-1:M,1);
local_Psiref = psiref(ids-1:M,1);
local_tref = tref(ids-1:M,1);
local_Vref = Vref(ids-1:M,1);


% If an abort is issued, the bike aborts the pre-defined reference and
% follow the abort-reference instead
if(abort)
    [local_Xref,local_Yref,local_Psiref] = genAbortTraj(est(1),est(2),est(3),Ns);
end

end


function [x_ref,y_ref,psi_ref] = genAbortTraj(x_est,y_est,psi_est,N)


step = 0.1; %Step size
r  = 5;
%N = 50;

x_ref = zeros(N,1);
y_ref = zeros(N,1);
psi_ref = zeros(N,1);
x_ref(1) = x_est;
y_ref(1) = y_est;
psi_ref(1) = psi_est;

% CALCULATE CENTER OF CIRCLE 
offset_x = r * sin(-psi_est);
offset_y = r * cos(-psi_est);
x_center = x_est + offset_x;
y_center = y_est + offset_y;

i = 1;
for t = step:step:(N*step-1)
    i = i+1;
    x_ref(i) = r*sin(-t+pi-psi_est) + x_center;
    y_ref(i) = r*cos(-t+pi-psi_est) + y_center;
    psi_ref(i) = atan2(y_ref(i)-y_ref(i-1),x_ref(i)-x_ref(i-1));  
end

end
